simulink model "Experiment5_DoubleLoop_model"  (R2012b)
settings: Solver=ode1  StartTime=0.0  StopTime=simulink_time  FixedStep=step_size  RelTol=1e-3
values from neighbouring files (symbols this model uses):
  exp_model = 1    [model_ref.mat]
  Inner_loop_amp = 20    [model_input.mat]
undefined symbols (not defined in the file or in its folder): PID_inner, PID_outer, Plant_K, Plant_T1, Plant_T2, simulink_start_time
libraries: simulink x3
settings Model: Creator=Administrator  LastModifiedBy=Administrator

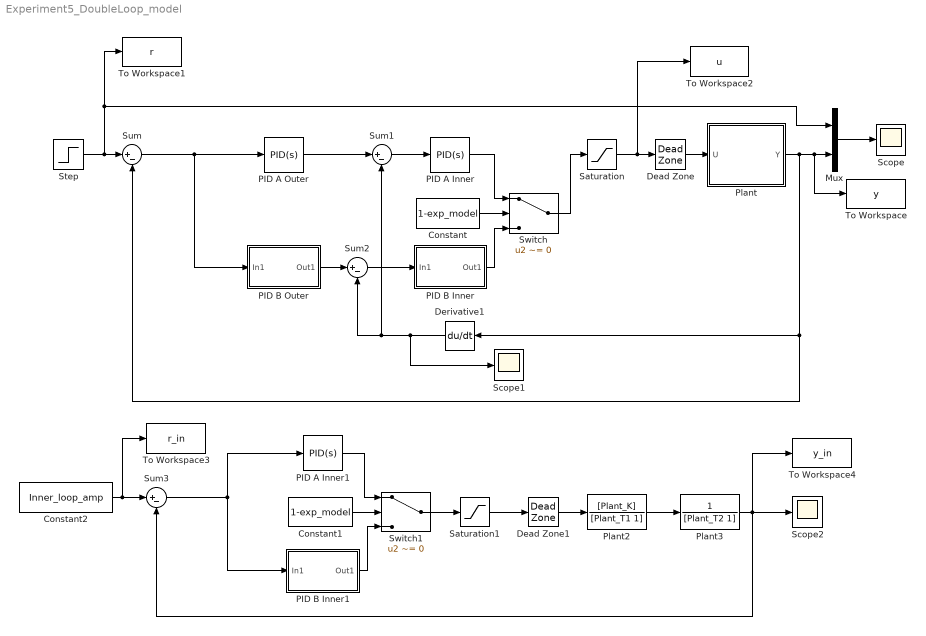
== system Experiment5_DoubleLoop_model ==
  Constant : Constant  Value=1-exp_model
  Constant1 : Constant  Value=1-exp_model
  Constant2 : Constant  Value=Inner_loop_amp
  Dead Zone : DeadZone  LowerValue=-2  UpperValue=2  SaturateOnIntegerOverflow=on
  Dead Zone1 : DeadZone  LowerValue=-2  UpperValue=2  SaturateOnIntegerOverflow=on
  Derivative1 : Derivative
  Mux : Mux  Inputs=2
  PID A Inner : simulink/Continuous/PID Controller  Controller=PID  TimeDomain=Continuous-time  SampleTime=0.002  IntegratorMethod=Trapezoidal  FilterMethod=Trapezoidal  Form=Parallel  P=PID_inner(1)  I=PID_inner(2)  D=PID_inner(3)  N=100  InitialConditionSource=internal  InitialConditionForIntegrator=0  InitialConditionForFilter=0  ExternalReset=none  LimitOutput=off  UpperSaturationLimit=inf  LowerSaturationLimit=-inf  LinearizeAsGain=on  AntiWindupMode=none  Kb=1  TrackingMode=off  Kt=1  PParamMin=[]  PParamMax=[]  IParamMin=[]  IParamMax=[]  DParamMin=[]  DParamMax=[]  NParamMin=[]  NParamMax=[]  KbParamMin=[]  KbParamMax=[]  KtParamMin=[]  KtParamMax=[]  POutMin=[]  POutMax=[]  IOutMin=[]  IOutMax=[]  DOutMin=[]  DOutMax=[]  NOutMin=[]  NOutMax=[]  KbOutMin=[]  KbOutMax=[]  KtOutMin=[]  KtOutMax=[]  IntegratorOutMin=[]  IntegratorOutMax=[]  FilterOutMin=[]  FilterOutMax=[]  SumOutMin=[]  SumOutMax=[]  SumI1OutMin=[]  SumI1OutMax=[]  SumI2OutMin=[]  SumI2OutMax=[]  SumI3OutMin=[]  SumI3OutMax=[]  SumDOutMin=[]  SumDOutMax=[]  SaturationOutMin=[]  SaturationOutMax=[]  IntegratorContinuousStateAttributes=''  IntegratorStateMustResolveToSignalObject=off  IntegratorRTWStateStorageClass=Auto  FilterContinuousStateAttributes=''  FilterStateMustResolveToSignalObject=off  FilterRTWStateStorageClass=Auto
  PID A Inner1 : simulink/Continuous/PID Controller  Controller=PID  TimeDomain=Continuous-time  SampleTime=0.002  IntegratorMethod=Trapezoidal  FilterMethod=Trapezoidal  Form=Parallel  P=PID_inner(1)  I=PID_inner(2)  D=PID_inner(3)  N=100  InitialConditionSource=internal  InitialConditionForIntegrator=0  InitialConditionForFilter=0  ExternalReset=none  LimitOutput=off  UpperSaturationLimit=inf  LowerSaturationLimit=-inf  LinearizeAsGain=on  AntiWindupMode=none  Kb=1  TrackingMode=off  Kt=1  PParamMin=[]  PParamMax=[]  IParamMin=[]  IParamMax=[]  DParamMin=[]  DParamMax=[]  NParamMin=[]  NParamMax=[]  KbParamMin=[]  KbParamMax=[]  KtParamMin=[]  KtParamMax=[]  POutMin=[]  POutMax=[]  IOutMin=[]  IOutMax=[]  DOutMin=[]  DOutMax=[]  NOutMin=[]  NOutMax=[]  KbOutMin=[]  KbOutMax=[]  KtOutMin=[]  KtOutMax=[]  IntegratorOutMin=[]  IntegratorOutMax=[]  FilterOutMin=[]  FilterOutMax=[]  SumOutMin=[]  SumOutMax=[]  SumI1OutMin=[]  SumI1OutMax=[]  SumI2OutMin=[]  SumI2OutMax=[]  SumI3OutMin=[]  SumI3OutMax=[]  SumDOutMin=[]  SumDOutMax=[]  SaturationOutMin=[]  SaturationOutMax=[]  IntegratorContinuousStateAttributes=''  IntegratorStateMustResolveToSignalObject=off  IntegratorRTWStateStorageClass=Auto  FilterContinuousStateAttributes=''  FilterStateMustResolveToSignalObject=off  FilterRTWStateStorageClass=Auto
  PID A Outer : simulink/Continuous/PID Controller  Controller=PID  TimeDomain=Continuous-time  SampleTime=0.002  IntegratorMethod=Trapezoidal  FilterMethod=Trapezoidal  Form=Parallel  P=PID_outer(1)  I=PID_outer(2)  D=PID_outer(3)  N=100  InitialConditionSource=internal  InitialConditionForIntegrator=0  InitialConditionForFilter=0  ExternalReset=none  LimitOutput=off  UpperSaturationLimit=inf  LowerSaturationLimit=-inf  LinearizeAsGain=on  AntiWindupMode=none  Kb=1  TrackingMode=off  Kt=1  PParamMin=[]  PParamMax=[]  IParamMin=[]  IParamMax=[]  DParamMin=[]  DParamMax=[]  NParamMin=[]  NParamMax=[]  KbParamMin=[]  KbParamMax=[]  KtParamMin=[]  KtParamMax=[]  POutMin=[]  POutMax=[]  IOutMin=[]  IOutMax=[]  DOutMin=[]  DOutMax=[]  NOutMin=[]  NOutMax=[]  KbOutMin=[]  KbOutMax=[]  KtOutMin=[]  KtOutMax=[]  IntegratorOutMin=[]  IntegratorOutMax=[]  FilterOutMin=[]  FilterOutMax=[]  SumOutMin=[]  SumOutMax=[]  SumI1OutMin=[]  SumI1OutMax=[]  SumI2OutMin=[]  SumI2OutMax=[]  SumI3OutMin=[]  SumI3OutMax=[]  SumDOutMin=[]  SumDOutMax=[]  SaturationOutMin=[]  SaturationOutMax=[]  IntegratorContinuousStateAttributes=''  IntegratorStateMustResolveToSignalObject=off  IntegratorRTWStateStorageClass=Auto  FilterContinuousStateAttributes=''  FilterStateMustResolveToSignalObject=off  FilterRTWStateStorageClass=Auto
  PID B Inner : Subsystem
  PID B Inner1 : Subsystem
  PID B Outer : Subsystem
  Plant : Subsystem
  Plant2 : TransferFcn  Numerator=[Plant_K]  Denominator=[Plant_T1 1]
  Plant3 : TransferFcn  Denominator=[Plant_T2 1]
  Saturation : Saturate  UpperLimit=19.2  LowerLimit=-19.2
  Saturation1 : Saturate  UpperLimit=19.2  LowerLimit=-19.2
  Scope : Scope
  Scope1 : Scope
  Scope2 : Scope
      settings: SaveName=ScopeData2
  Step : Step  Time=simulink_start_time  After=60  SampleTime=0
  Sum{,1..3} (4 alike) : Sum  Inputs=|+-
  Switch : Switch  Criteria=u2 ~= 0
  Switch1 : Switch  Criteria=u2 ~= 0
  To Workspace : ToWorkspace  VariableName=y  SampleTime=-1
  To Workspace1 : ToWorkspace  VariableName=r  SampleTime=-1
  To Workspace2 : ToWorkspace  VariableName=u  SampleTime=-1
  To Workspace3 : ToWorkspace  VariableName=r_in  SampleTime=-1
  To Workspace4 : ToWorkspace  VariableName=y_in  SampleTime=-1
  wires:
  Step/1 -> Mux/1, To Workspace1/1, Sum/1
  Mux/1 -> Scope/1
  Saturation/1 -> To Workspace2/1, Dead Zone/1
  Plant/1(Y) -> To Workspace/1, Mux/2, Derivative1/1, Sum/2
  Dead Zone/1 -> Plant/1(U)
  PID A Outer/1 -> Sum1/1
  Sum1/1 -> PID A Inner/1
  PID B Outer/1(Out1) -> Sum2/1
  Sum2/1 -> PID B Inner/1(In1)
  Derivative1/1 -> Scope1/1, Sum2/2, Sum1/2
  Sum/1 -> PID B Outer/1(In1), PID A Outer/1
  Switch/1 -> Saturation/1
  PID A Inner/1 -> Switch/1
  PID B Inner/1(Out1) -> Switch/3
  Constant/1 -> Switch/2
  Saturation1/1 -> Dead Zone1/1
  Dead Zone1/1 -> Plant2/1
  Sum3/1 -> PID A Inner1/1, PID B Inner1/1(In1)
  Switch1/1 -> Saturation1/1
  PID A Inner1/1 -> Switch1/1
  PID B Inner1/1(Out1) -> Switch1/3
  Constant1/1 -> Switch1/2
  Plant2/1 -> Plant3/1
  Constant2/1 -> To Workspace3/1, Sum3/1
  Plant3/1 -> To Workspace4/1, Scope2/1, Sum3/2

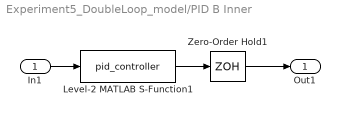
== system Experiment5_DoubleLoop_model/PID B Inner ==
  In1 : Inport
  Level-2 MATLAB S-Function1 : M-S-Function  FunctionName=pid_controller  Parameters=PID_inner(1),PID_inner(2),PID_inner(3)
  Zero-Order Hold1 : ZeroOrderHold  SampleTime=-1
  Out1 : Outport
  wires:
  In1/1 -> Level-2 MATLAB S-Function1/1
  Level-2 MATLAB S-Function1/1 -> Zero-Order Hold1/1
  Zero-Order Hold1/1 -> Out1/1

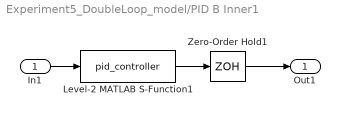
== system Experiment5_DoubleLoop_model/PID B Inner1 ==
  In1 : Inport
  Level-2 MATLAB S-Function1 : M-S-Function  FunctionName=pid_controller  Parameters=PID_inner(1),PID_inner(2),PID_inner(3)
  Zero-Order Hold1 : ZeroOrderHold  SampleTime=-1
  Out1 : Outport
  wires:
  In1/1 -> Level-2 MATLAB S-Function1/1
  Level-2 MATLAB S-Function1/1 -> Zero-Order Hold1/1
  Zero-Order Hold1/1 -> Out1/1

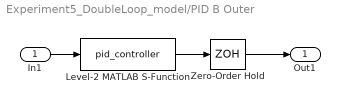
== system Experiment5_DoubleLoop_model/PID B Outer ==
  In1 : Inport
  Level-2 MATLAB S-Function : M-S-Function  FunctionName=pid_controller  Parameters=PID_outer(1),PID_outer(2),PID_outer(3)
  Zero-Order Hold : ZeroOrderHold  SampleTime=-1
  Out1 : Outport
  wires:
  Zero-Order Hold/1 -> Out1/1
  In1/1 -> Level-2 MATLAB S-Function/1
  Level-2 MATLAB S-Function/1 -> Zero-Order Hold/1

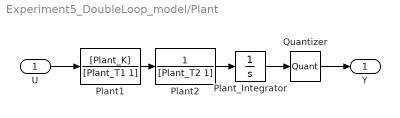
== system Experiment5_DoubleLoop_model/Plant ==
  U : Inport
  Plant1 : TransferFcn  Numerator=[Plant_K]  Denominator=[Plant_T1 1]
  Plant2 : TransferFcn  Denominator=[Plant_T2 1]
  Plant_Integrator : Integrator
  Quantizer : Quantizer  QuantizationInterval=0.005
  Y : Outport
  wires:
  U/1 -> Plant1/1
  Quantizer/1 -> Y/1
  Plant1/1 -> Plant2/1
  Plant_Integrator/1 -> Quantizer/1
  Plant2/1 -> Plant_Integrator/1
